simulink model "testing"  (R2023a)
settings: Solver=VariableStepAuto  StartTime=0.0  StopTime=inf  RelTol=1e-3
libraries: commdigbbndpm3 x1, commrandsrc3 x1, hdlsllib x1
settings Model: Creator=acer  LastModifiedBy=acer
settings OptimizationCC: BlockReduction=off  ConditionallyExecuteInputs=off

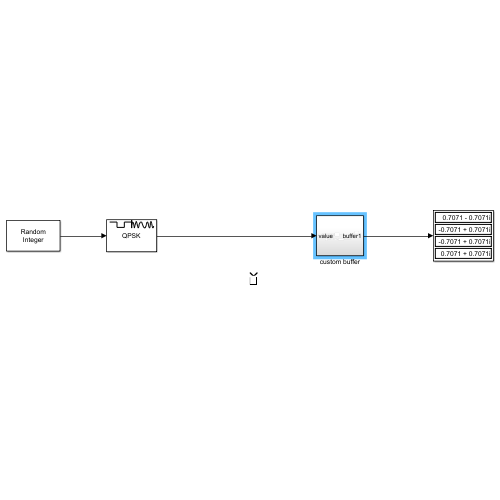
[thumbnail: Simulink's stored preview of the top-level diagram]
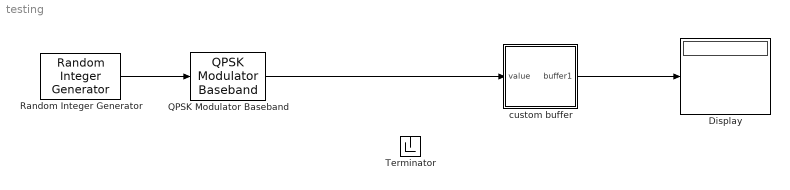
== system testing ==
  Display : Display
  QPSK Modulator Baseband : commdigbbndpm3/QPSK Modulator Baseband  InType=Integer  Enc=Gray  Ph=pi/4  outDtype=Fixed-point  outWordLen=16  outUDDataType=sfix(16)  outFracLenMode=Best precision  outFracLen=15  outDataTypeStr=fixdt(1,16)  outLastDataTypeStr=fixdt(1,16)
      settings: LibrarySourceBlock=|
      | commhdldigbbndpm/QPSK
      | Modulator
      | Baseband
  Random Integer Generator : commrandsrc3/Random Integer Generator  SetSize=4  SeedSource=Auto  Seed=0  SampleTime=1  SamplesPerFrame=1  OutputDataType=uint8  SimulateUsing=Interpreted execution
  Terminator : Terminator
  custom buffer : Subsystem
  wires:
  custom buffer/1(buffer1) -> Display/1
  Random Integer Generator/1 -> QPSK Modulator Baseband/1
  QPSK Modulator Baseband/1 -> custom buffer/1(value)

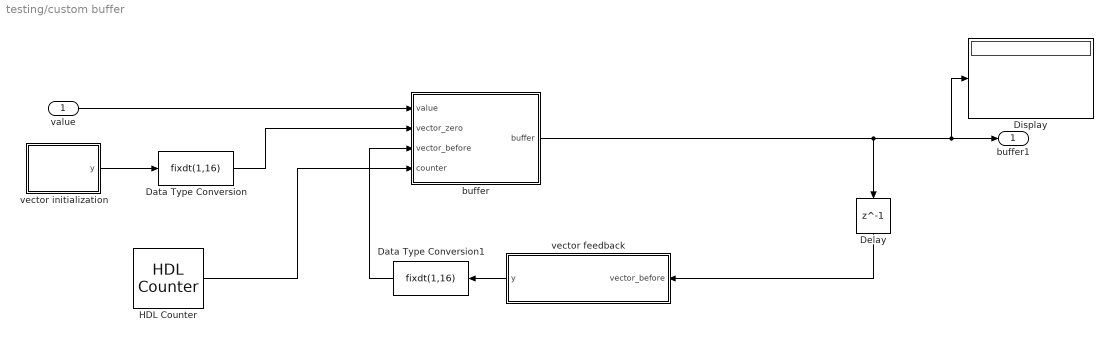
== system testing/custom buffer ==
  value : Inport
  Data Type Conversion : DataTypeConversion  OutMin=0  OutMax=1  OutDataTypeStr=fixdt(1,16)  SaturateOnIntegerOverflow=off  RndMeth=Floor
  Data Type Conversion1 : DataTypeConversion  OutMin=0  OutMax=1  OutDataTypeStr=fixdt(1,16)  SaturateOnIntegerOverflow=off  RndMeth=Floor
  Delay : Delay  DelayLength=1
  Display : Display
  HDL Counter : hdlsllib/Sources/HDL Counter  CountType=Count limited  CountInit=1  CountStep=1  CountMax=4  CountFromType=Initial value  CountFrom=1  CountResetPort=off  CountLoadPort=off  CountEnbPort=off  CountDirPort=off  CountHitOutputPort=off  CountDataType=Unsigned  CountWordLen=8  CountFracLen=0  CountSampTime=1
  buffer : MATLAB Function  TreatAsAtomicUnit=on
  vector feedback : MATLAB Function  TreatAsAtomicUnit=on
  vector initialization : MATLAB Function  TreatAsAtomicUnit=on
  buffer1 : Outport
  wires:
  HDL Counter/1 -> buffer/4(counter)
  value/1 -> buffer/1(value)
  vector initialization/1(y) -> Data Type Conversion/1
  Data Type Conversion/1 -> buffer/2(vector_zero)
  buffer/1(buffer) -> Delay/1, Display/1, buffer1/1
  Delay/1 -> vector feedback/1(vector_before)
  vector feedback/1(y) -> Data Type Conversion1/1
  Data Type Conversion1/1 -> buffer/3(vector_before)

== matlab function testing/custom buffer/buffer ==
  data: value input; vector_zero input; vector_before input; counter input; buffer output
function buffer = fcn(value, vector_zero, vector_before, counter)
%#codegen
if(counter == 0)
    buffer = vector_zero;
else
    buffer = vector_before;
end

buffer(counter) = value;

== matlab function testing/custom buffer/vector initialization ==
  data: y output
function y = fcn()
%#codegen

y = complex(ones(1,4));

== matlab function testing/custom buffer/vector feedback ==
  data: y output; vector_before input
function y = fcn(vector_before)
%#codegen

y = complex(vector_before);
